simulink model "line_follower"  (R2020a)
settings: Solver=ode4  StartTime=0.0  StopTime=10.0  FixedStep=0.1  RelTol=1e-3
values from neighbouring files (symbols this model uses):
  a = 1    [mobile_robots.m]
  b = -2    [mobile_robots.m]
  b0 = 1/2    (= 0.5)    [mobile_robots.m]
  b1 = 2    [mobile_robots.m]
  c = 4    [mobile_robots.m]
  kp1 = 0.5    [mobile_robots.m]
  kp2 = 1    [mobile_robots.m]
  L = 1    [mobile_robots.m]
  speed = 10    [mobile_robots.m]
  theta_start = theta(i)    [mobile_robots.m]
  x_start = x(i)    [mobile_robots.m]
  y_start = y(i)    [mobile_robots.m]
settings Model: Creator=krzysztof  LastModifiedBy=krzysztof

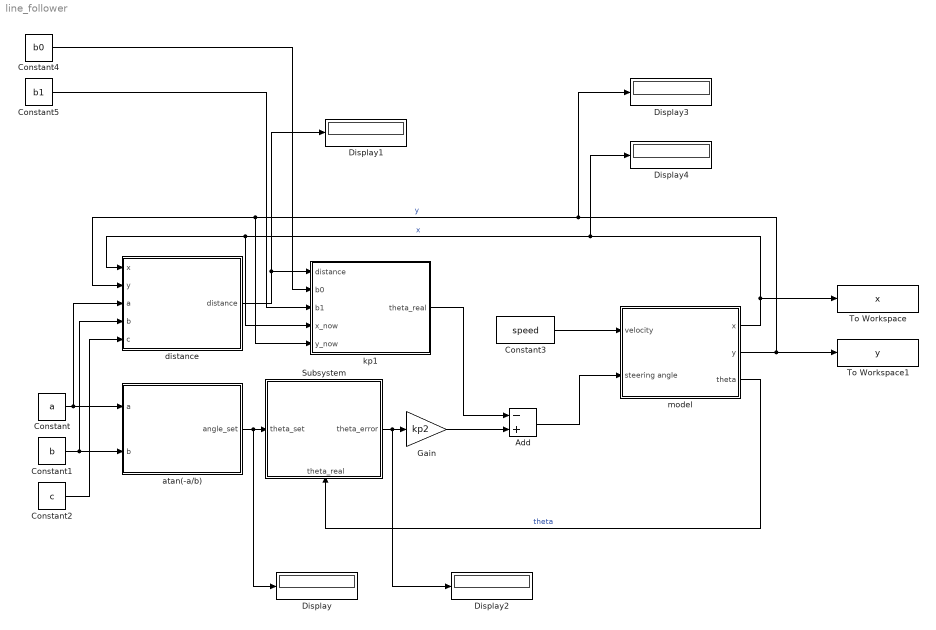
== system line_follower ==
  Add : Sum  Inputs=-+
  Constant : Constant  Value=a
  Constant1 : Constant  Value=b
  Constant2 : Constant  Value=c
  Constant3 : Constant  Value=speed
  Constant4 : Constant  Value=b0
  Constant5 : Constant  Value=b1
  Display{,1..4} (5 alike) : Display
  Gain : Gain  Gain=kp2
  Subsystem : Subsystem
      settings: PortSchema="{\"entries\":[{\"content\":{\"sides\":[{\"content\":{\"connectorIds\":[\"In1\"]},\"type\":\"ConnectorPlacement.EquallySpacedRectSide\",\"uuid\":\"fc3d2d42-6b75-4455-93d0-24c477eba1e2\"},{\"content\":{\"connectorIds\":[\"Out1\"],\"side\":\"RIGHT\"},\"type\":\"ConnectorPlacement.EquallySpacedRectSide\",\"uuid\":\"640ab7b6-8e5c-42d1-9d7a-31c2e9c3df8c\"},{\"content\":{\"connectorIds\":[],\"side\":\"TOP\"},\"type\":\"ConnectorPlacement.EquallySpacedRectSide\",\"uuid\":\"7c89bff5-0cce-42ff-a4c1-7cad39dc7ecc\"},{\"content\":{\"connectorIds\":[\"In2\"],\"side\":\"BOTTOM\"},\"type\":\"ConnectorPlacement.EquallySpacedRectSide\",\"uuid\":\"a37ec459-fa6b-4142-b403-d1bf8803b979\"}]},\"type\":\"ConnectorPlacement.EquallySpacedConnector\",\"uuid\":\"f605075b-9a69-4b03-9ecf-c2f7e2b5f79a\"}],\"packageUris\":[\"http://schema.mathworks.com/mf0/Connector/19700101\"],\"version\":\"1.0\"}"
  To Workspace : ToWorkspace  VariableName=x  SampleTime=-1
      settings: Save2DSignal=2-D array (concatenate along first dimension)
  To Workspace1 : ToWorkspace  VariableName=y  SampleTime=-1
      settings: Save2DSignal=2-D array (concatenate along first dimension)
  atan(-a/b) : Subsystem
  distance : Subsystem
  kp1 : Subsystem
  model : Subsystem
  wires:
  Constant/1 -> distance/3(a), atan(-a/b)/1(a)
  Constant1/1 -> distance/4(b), atan(-a/b)/2(b)
  Constant3/1 -> model/1(velocity)
  distance/1(distance) -> kp1/1(distance), Display1/1
  atan(-a/b)/1(angle_set) -> Display/1, Subsystem/1(theta_set)
  Subsystem/1(theta_error) -> Display2/1, Gain/1
  model/3(theta) -> Subsystem/2(theta_real)  "theta"
  Constant2/1 -> distance/5(c)
  model/1(x) -> To Workspace/1, Display4/1, kp1/4(x_now), distance/1(x)  "x"
  model/2(y) -> To Workspace1/1, Display3/1, kp1/5(y_now), distance/2(y)  "y"
  Add/1 -> model/2(steering angle)
  Gain/1 -> Add/2
  kp1/1(theta_real) -> Add/1
  Constant5/1 -> kp1/3(b1)
  Constant4/1 -> kp1/2(b0)

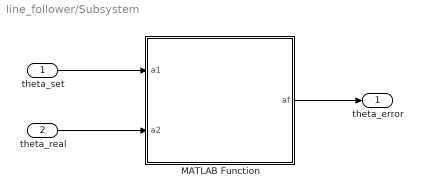
== system line_follower/Subsystem ==
  theta_set : Inport
  theta_real : Inport  Port=2
  MATLAB Function : MATLAB Function  TreatAsAtomicUnit=on
  theta_error : Outport
  wires:
  MATLAB Function/1(af) -> theta_error/1
  theta_set/1 -> MATLAB Function/1(a1)
  theta_real/1 -> MATLAB Function/2(a2)

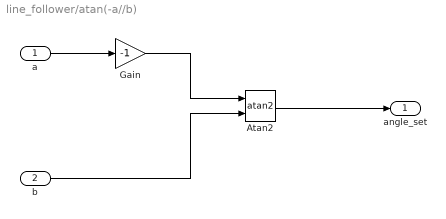
== system line_follower/atan(-a//b) ==
  a : Inport
  b : Inport  Port=2
  Atan2 : Trigonometry  Operator=atan2  OutputSignalType=real
  Gain : Gain  Gain=-1
  angle_set : Outport
  wires:
  a/1 -> Gain/1
  Gain/1 -> Atan2/1
  b/1 -> Atan2/2
  Atan2/1 -> angle_set/1

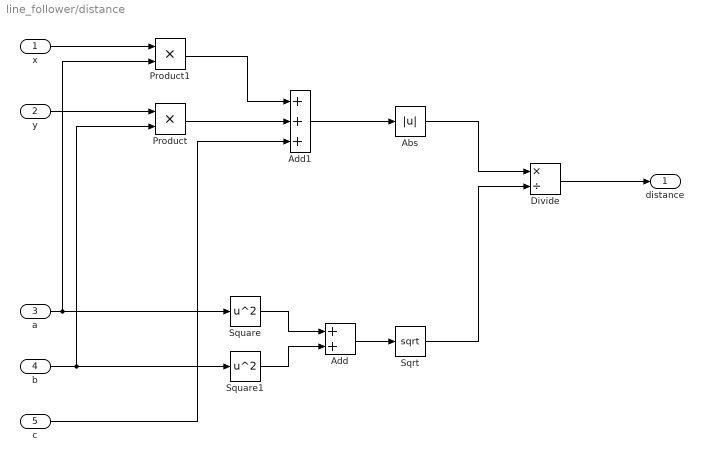
== system line_follower/distance ==
  x : Inport
  y : Inport  Port=2
  a : Inport  Port=3
  b : Inport  Port=4
  c : Inport  Port=5
  Abs : Abs
  Add : Sum
  Add1 : Sum  Inputs=+++
  Divide : Product  Inputs=*/
  Product : Product
  Product1 : Product
  Sqrt : Sqrt  SaturateOnIntegerOverflow=on
  Square : Math  Operator=square  SaturateOnIntegerOverflow=on
  Square1 : Math  Operator=square  SaturateOnIntegerOverflow=on
  distance : Outport
  wires:
  a/1 -> Product1/2, Square/1
  b/1 -> Product/2, Square1/1
  Square/1 -> Add/1
  Square1/1 -> Add/2
  Add/1 -> Sqrt/1
  Divide/1 -> distance/1
  Sqrt/1 -> Divide/2
  Abs/1 -> Divide/1
  y/1 -> Product/1
  x/1 -> Product1/1
  Add1/1 -> Abs/1
  Product1/1 -> Add1/1
  Product/1 -> Add1/2
  c/1 -> Add1/3

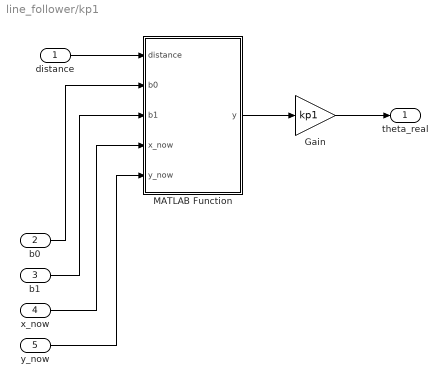
== system line_follower/kp1 ==
  distance : Inport
  b0 : Inport  Port=2
  b1 : Inport  Port=3
  x_now : Inport  Port=4
  y_now : Inport  Port=5
  Gain : Gain  Gain=kp1
  MATLAB Function : MATLAB Function  TreatAsAtomicUnit=on
  theta_real : Outport
  wires:
  distance/1 -> MATLAB Function/1(distance)
  Gain/1 -> theta_real/1
  MATLAB Function/1(y) -> Gain/1
  b0/1 -> MATLAB Function/2(b0)
  b1/1 -> MATLAB Function/3(b1)
  x_now/1 -> MATLAB Function/4(x_now)
  y_now/1 -> MATLAB Function/5(y_now)

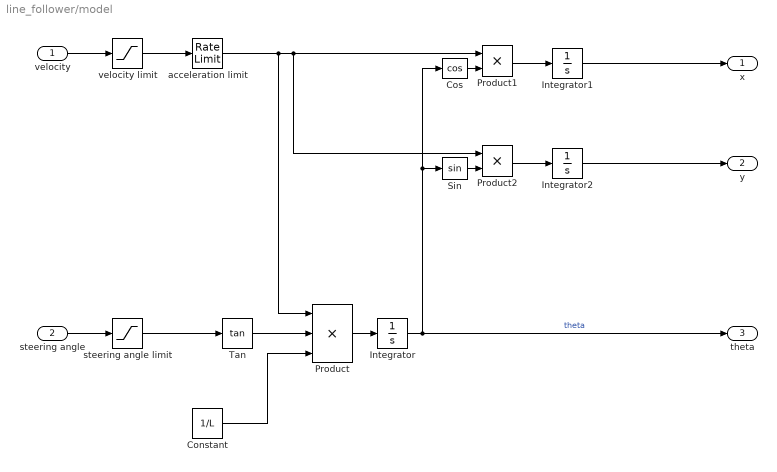
== system line_follower/model ==
  velocity : Inport
  steering angle : Inport  Port=2
  Constant : Constant  Value=1/L
  Cos : Trigonometry  Operator=cos  OutputSignalType=real
  Integrator : Integrator  InitialCondition=theta_start
  Integrator1 : Integrator  InitialCondition=x_start
  Integrator2 : Integrator  InitialCondition=y_start
  Product : Product  Inputs=3
  Product1 : Product
  Product2 : Product
  Sin : Trigonometry  OutputSignalType=real
  Tan : Trigonometry  Operator=tan  OutputSignalType=real
  acceleration limit : RateLimiter  SampleTimeMode=inherited
  steering angle limit : Saturate  UpperLimit=1  LowerLimit=-1  LinearizeAsGain=off
  velocity limit : Saturate  UpperLimit=2  LowerLimit=-2
  x : Outport
  y : Outport  Port=2
  theta : Outport  Port=3
  wires:
  Product1/1 -> Integrator1/1
  Integrator2/1 -> y/1
  Product2/1 -> Integrator2/1
  Integrator/1 -> theta/1, Cos/1, Sin/1  "theta"
  Integrator1/1 -> x/1
  Cos/1 -> Product1/2
  Tan/1 -> Product/2
  Constant/1 -> Product/3
  steering angle limit/1 -> Tan/1
  acceleration limit/1 -> Product/1, Product2/1, Product1/1
  Sin/1 -> Product2/2
  Product/1 -> Integrator/1
  steering angle/1 -> steering angle limit/1
  velocity limit/1 -> acceleration limit/1
  velocity/1 -> velocity limit/1

== matlab function line_follower/Subsystem/MATLAB Function ==
  data: a1 input; af output; a2 input
function af=angdif2(a1,a2)   % radians angles version
%
%   input : a1, a2
% output: af
a3=mod(a1-a2,2*pi);
af= 0;
q1=pi/2;
q2=pi;
q3=3*pi/2;
q4=2*pi;

if (0<a3)&&(a3<=q1)
    af=a3;
elseif (q1<a3)&&(a3<=q2) 
     af=a3;
elseif (q2<a3)&&(a3<=q3) 
    af=a3-q4;
elseif (q3<a3)&&(a3<=q4) 
    af= a3-q4;
elseif (-q1<=a3)&&(a3<0)    
    af=a3;
elseif (-q2<=a3)&&(a3<-q1) 
    af=a3;
elseif (-q3<=a3)&&(a3<-q2) 
    af =q4+a3;
elseif (-q4<=a3)&&(a3<-q3)
    af = q4+a3;
end

if af==pi 
    af=-pi;
end

return

== matlab function line_follower/kp1/MATLAB Function ==
  data: distance input; y output; b0 input; b1 input; x_now input; y_now input
function y = fcn(distance, b0, b1, x_now, y_now)

    f = @(x) b0*x+b1;

    if y_now > f(x_now)
        distance = distance * (-1);
    end

y = distance;
